simulink model "Res_Angle_Filter"  (Simulink 7.6)
settings: Solver=ode45  StartTime=0.0  StopTime=0.02  RelTol=1e-3
settings Model: Creator=Vano  LastModifiedBy=Vano

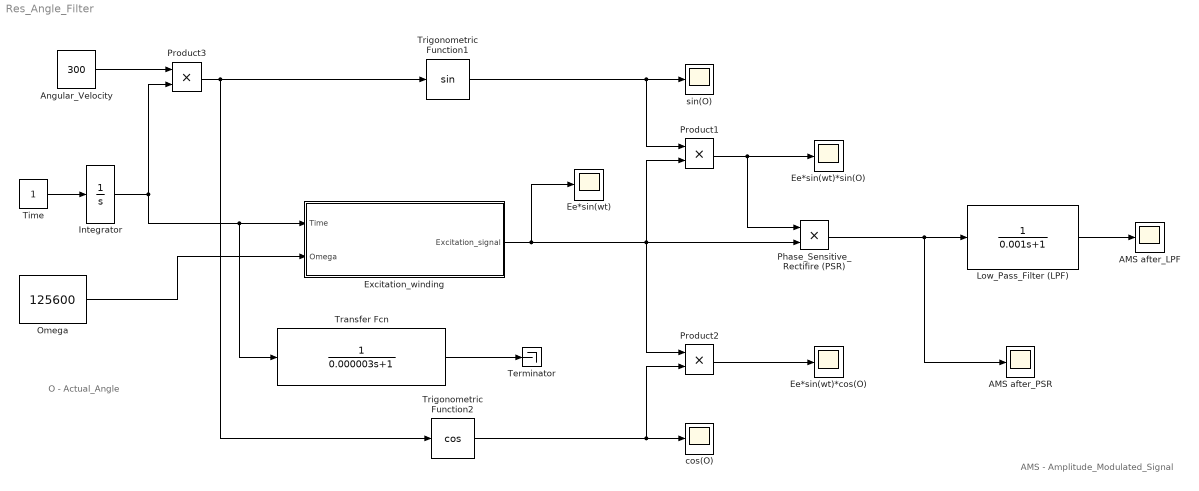
== system Res_Angle_Filter ==
  note: O - Actual_Angle
  note: AMS - Amplitude_Modulated_Signal
  AMS after_LPF : Scope
      settings: SaveName=ScopeData6
  AMS after_PSR : Scope
      settings: SaveName=ScopeData7
  Angular_Velocity : Constant  Value=300
  Ee*sin(wt) : Scope
      settings: YMin=-1  YMax=1  SaveName=ScopeData2
  Ee*sin(wt)*cos(O) : Scope
      settings: SaveName=ScopeData3
  Ee*sin(wt)*sin(O) : Scope
      settings: YMin=-0.03  YMax=0.03
  Excitation_winding : Subsystem
  Integrator : Integrator
  Low_Pass_Filter (LPF) : TransferFcn  Denominator=[0.001 1]
  Omega : Constant  Value=125600
  Phase_Sensitive_Rectifire (PSR) : Product  RndMeth=Zero
  Product1 : Product  RndMeth=Zero
  Product2 : Product  RndMeth=Zero
  Product3 : Product  RndMeth=Zero
  Terminator : Terminator
  Time : Constant
  Transfer Fcn : TransferFcn  Denominator=[0.000003 1]
  Trigonometric Function1 : Trigonometry
  Trigonometric Function2 : Trigonometry  Operator=cos
  cos(O) : Scope
      settings: SaveName=ScopeData4
  sin(O) : Scope
  wires:
  Time/1 -> Integrator/1
  Omega/1 -> Excitation_winding/2(Omega)
  Integrator/1 -> Transfer Fcn/1, Excitation_winding/1(Time), Product3/2
  Trigonometric Function1/1 -> sin(O)/1, Product1/1
  Excitation_winding/1(Excitation_signal) -> Ee*sin(wt)/1, Product1/2, Product2/1, Phase_Sensitive_Rectifire (PSR)/2
  Trigonometric Function2/1 -> Product2/2, cos(O)/1
  Product1/1 -> Phase_Sensitive_Rectifire (PSR)/1, Ee*sin(wt)*sin(O)/1
  Product2/1 -> Ee*sin(wt)*cos(O)/1
  Transfer Fcn/1 -> Terminator/1
  Angular_Velocity/1 -> Product3/1
  Product3/1 -> Trigonometric Function1/1, Trigonometric Function2/1
  Phase_Sensitive_Rectifire (PSR)/1 -> Low_Pass_Filter (LPF)/1, AMS after_PSR/1
  Low_Pass_Filter (LPF)/1 -> AMS after_LPF/1

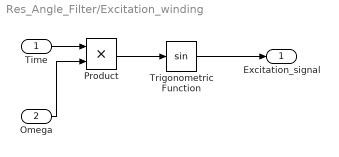
== system Res_Angle_Filter/Excitation_winding ==
  Time : Inport
  Omega : Inport  Port=2
  Product : Product  RndMeth=Zero
  Trigonometric Function : Trigonometry
  Excitation_signal : Outport
  wires:
  Product/1 -> Trigonometric Function/1
  Time/1 -> Product/1
  Trigonometric Function/1 -> Excitation_signal/1
  Omega/1 -> Product/2
